simulink model "DCDC_SEPIC_TopLevelModel"  (R2024b)
settings: configuration reference "ConfigSet_ode23t_TopLevel" (kept outside this file)
undefined symbols (not defined in the file): psu_V, ts10ms, ts500us
libraries: fl_lib x21, ee_lib x9, dspstat3 x8, nesl_utility x7, simulink x3, batteryecm_lib x3, SEPIC_utilities x1
settings Model: DataDictionary=LocalDataD_TopLevelModelData.sldd  SILPILSystemUnderTest=refmodels  ExtModeTrigDuration=8  Creator=vivekr  LastModifiedBy=vlenzi
settings ConfigSetRef: SourceName=ConfigSet_ode23t_TopLevel

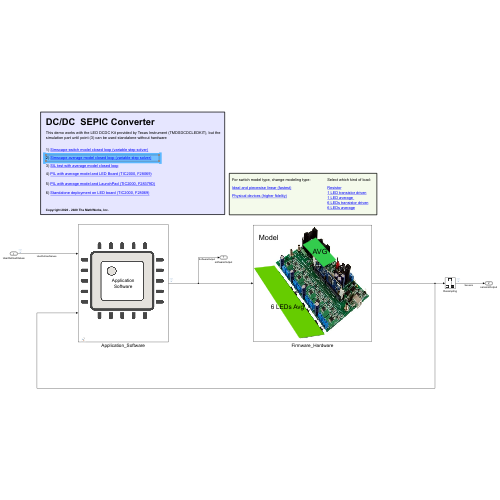
[thumbnail: Simulink's stored preview of the top-level diagram]
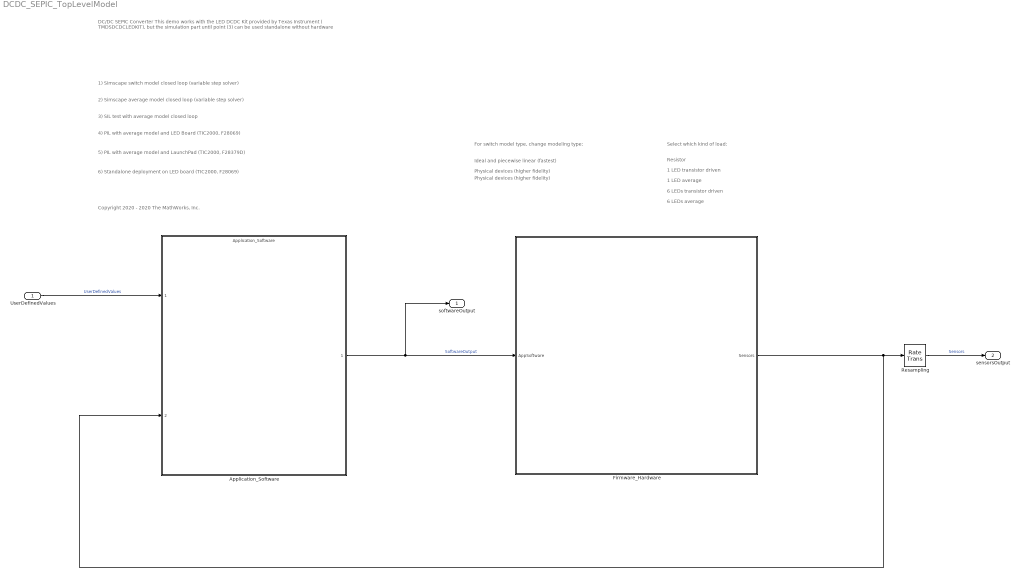
== system DCDC_SEPIC_TopLevelModel ==
  note: Copyright 2020 - 2020 The MathWorks, Inc.
  note: Ideal and piecewise linear (fastest)
  note: DC/DC SEPIC Converter
      |
      | This demo works with the LED DCDC Kit provided by Texas Instrument ( TMDSDCDCLEDKIT), but the simulation part until point (3) can be used standalone without hardware
  note: 6) Standalone deployment on LED board (TIC2000, F28069)
  note: 2) Simscape average model closed loop (variable step solver)
  note: 1) Simscape switch model closed loop (variable step solver)
  note: Physical devices (higher fidelity)
  note: For switch model type, change modeling type:
  note: 3) SIL test with average model closed loop
  note: Select which kind of load:
  note: Resistor
  note: 1 LED transistor driven
  note: 1 LED average
  note: 6 LEDs transistor driven
  note: 6 LEDs average
  note: 4) PIL with average model and LED Board (TIC2000, F28069)
  note: Physical devices (higher fidelity)
  note: 5) PIL with average model and LaunchPad (TIC2000, F28379D)
  UserDefinedValues : Inport  OutDataTypeStr=Bus: UserDefinedValues  Interpolate=off
  Application_Software : ModelReference  ModelNameDialog=Application_Software  SimulationMode=Normal  ModelReferenceVersion=9.13
      mask Display: image('cpu.png');disp('Application\nSoftware');
  Firmware_Hardware : Subsystem
      mask Display: image('SEPIC_converter_TI_Kit.jpg');patch([0.42 0.53 0.7 0.595],[0.83 0.89 0.7 0.64], [0.2 0.8 0.3]);text(0.505,0.78,'\fontsize{28}AVG','texmode', 'on');text(0.05,0.9,'\fontsize{28}Model','texmode', 'on');patch([0.39 0.01 0.18 0.6],[0.03 0.63 0.65 0.06], [0.4 0.8 0]);text(0.15,0.3,'\fontsize{25}6 LEDs Avg','texmode', 'on');
  Resampling : RateTransition  OutPortSampleTime=ts500us
  softwareOutput : Outport  OutDataTypeStr=Bus: AppSoftware
  sensorsOutput : Outport  Port=2  OutDataTypeStr=Bus: Sensors
  wires:
  Application_Software/1 -> Firmware_Hardware/1(AppSoftware), softwareOutput/1  "SoftwareOutput"
  Firmware_Hardware/1(Sensors) -> Resampling/1, Application_Software/2
  UserDefinedValues/1 -> Application_Software/1  "UserDefinedValues"
  Resampling/1 -> sensorsOutput/1  "Sensors"

== system DCDC_SEPIC_TopLevelModel/Firmware_Hardware ==
  Bus Element In : Inport  PortName=AppSoftware  Element=dcpwmSEPIC
  Bus Element In1 : Inport  PortName=AppSoftware  Element=dcpwmLEDvector
  Hardware_Filter : Subsystem  Variant=on  VariantControl=Variant1  AllowZeroVariantControls=on
  Bus Element Out : Outport  PortName=Sensors  Element=voltSEPIC
  Bus Element Out1 : Outport  PortName=Sensors  Element=currSEPIC
  Bus Element Out2 : Outport  PortName=Sensors  Element=currLEDstrips
  Bus Element Out3 : Outport  PortName=Sensors  Element=voltPSU
  wires:
  Hardware_Filter/2(currSEPIC) -> Bus Element Out1/1  "currSEPIC"
  Hardware_Filter/3(currLEDstrips) -> Bus Element Out2/1  "currLEDstrips"
  Bus Element In1/1 -> Hardware_Filter/2(dcpwmLEDvector)
  Hardware_Filter/4(voltPSU) -> Bus Element Out3/1  "voltPSU"
  Hardware_Filter/1(voltSEPIC) -> Bus Element Out/1  "voltSEPIC"
  Bus Element In/1 -> Hardware_Filter/1(dcpwmSEPIC)

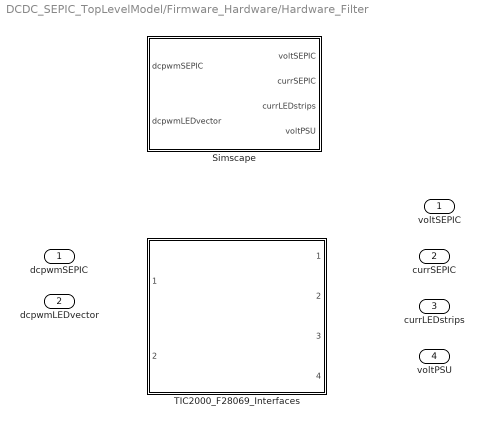
== system DCDC_SEPIC_TopLevelModel/Firmware_Hardware/Hardware_Filter ==
  dcpwmSEPIC : Inport  Unit=1
  dcpwmLEDvector : Inport  Port=2  Unit=1
  Simscape : Subsystem  VariantControl=Var_Plant==0
  TIC2000_F28069_Interfaces : Subsystem  VariantControl=Var_Plant ==1  ReferencedSubsystem=TIC2000_F28069_Interfaces
      settings: PermitHierarchicalResolution=None
  voltSEPIC : Outport  Unit=V  VectorParamsAs1DForOutWhenUnconnected=off
  currSEPIC : Outport  Port=2  Unit=mA  VectorParamsAs1DForOutWhenUnconnected=off
  currLEDstrips : Outport  Port=3  Unit=mA  PortDimensions=6  VectorParamsAs1DForOutWhenUnconnected=off
  voltPSU : Outport  Port=4  Unit=V  VectorParamsAs1DForOutWhenUnconnected=off

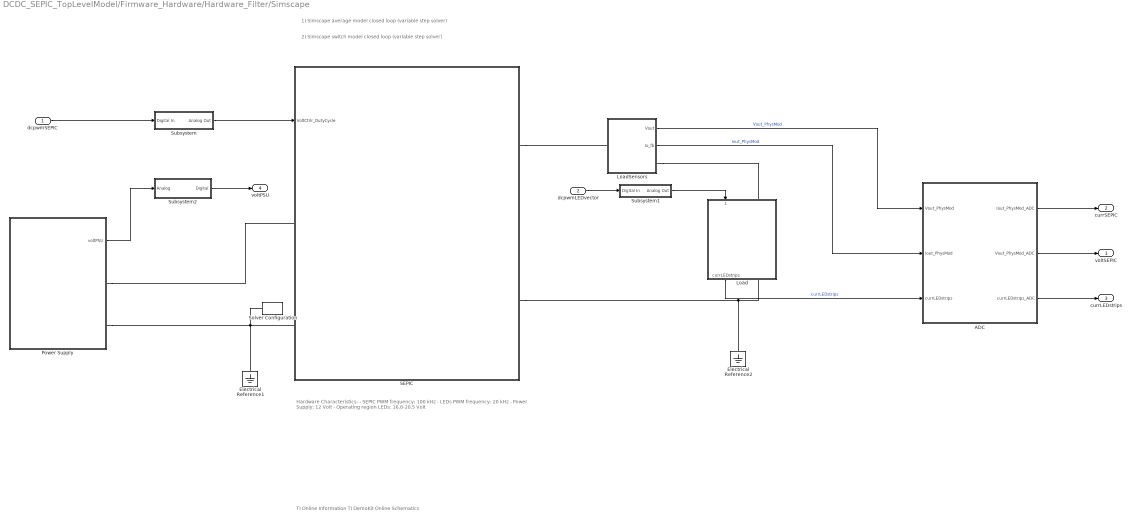
== system DCDC_SEPIC_TopLevelModel/Firmware_Hardware/Hardware_Filter/Simscape ==
  note: Hardware Characteristics:
      | - SEPIC PWM frequency: 100 kHz
      | - LEDs PWM frequency: 20 kHz
      | - Power Supply: 12 Volt
      | - Operating region LEDs: 16.8-20.5 Volt
  note: 2) Simscape switch model closed loop (variable step solver)
  note: 1) Simscape average model closed loop (variable step solver)
  note: TI Online Information
      | TI DemoKit Online Schematics
  dcpwmSEPIC : Inport  OutDataTypeStr=single  Unit=1  PortDimensions=1
  dcpwmLEDvector : Inport  Port=2  Unit=1
  ADC : Subsystem
      mask Display: disp('ADC');
  Electrical Reference1 : fl_lib/Electrical/Electrical Elements/Electrical Reference
  Electrical Reference2 : fl_lib/Electrical/Electrical Elements/Electrical Reference
  Load : Subsystem  Variant=on  VariantControlMode=label  VariantControl=Variant1  LabelModeActiveChoice=SixLEDStripsAvg
      mask Display: image('LED_Picture.jpg'); % Use "Edit Image" on toolstrip to change.
  LoadSensors : Subsystem
  Power Supply : Subsystem  Variant=on  VariantControlMode=label  VariantControl=Variant1  LabelModeActiveChoice=PowerSupply
      mask Display:
      | % Plot points to set plot range
      | color('white');plot(1.5, 2.5);plot(-1.5, -2)
      | color('black');
      | % Battery icon
      | plot([0 0], [2.5 1.3])
      | plot([0 0], [-0.6 -1.6])
      | patch([-1 1 1 -1]*0.4, [1 1 -1 -1]*0.15+0.7,[0;0;0]);
      | patch([-1 1 1 -1]*0.4, [1 1 -1 -1]*0.15-0.6,[0;0;0]);
      | patch([-1 1 1 -1]*0.8, [1 1 -1 -1]*0.15+1.3,[0;0;0]);
      | patch([-1 1 1 -1]*0.8, [1 1 -1 -1]*0.15+0.0,[0;0;0]);
      | text(1.2, 0.25,'+');
      | text(1.2,-1.1,'_');
      | text(1.2,1.8,'m');
  SEPIC : Subsystem  Variant=on  VariantControl=Variant1
      mask Display: image('dc_dc_converter.png'); % Use "Edit Image" on toolstrip to change.
  Solver Configuration : nesl_utility/Solver Configuration  PhysicalDomain=network_engine_domain  SubClassName=solver  LeftPortType=input  RightPortType=generic  Tones=[]  Harmonics=[]  SimulateNoise=off  Profile=off  UseLocalSampling=off  EnableSwitchedLinearOptims=on  FrequencyDomain=off  UseCCode=off  RelTol=0.001  AbsTol=1e-06  MinStep=1e-09  ToWorkspace=off  RevertToSquareIcSolve=off  NumHomotopyIterations=100  PhasorMode=off  PhasorModeNumHarmonics=1  ConsistencySolver=NEWTON_XTOL_AFTER_FTOL  IndexReductionMethod=DerivativeReplacement  DoDC=off  ResidualTolerance=1e-9  ConsistencyTolSource=GLOBAL  ConsistencyAbsTol=0.001  ConsistencyRelTol=0.001  ConsistencyTolFactor=0.001  UseLocalSolver=off  LocalSolverChoice=NE_BACKWARD_EULER_ADVANCER  ResolveIndetEquations=on  FunctionEvalNumThread=1  LocalSolverSampleTime=2e-7  DoFixedCost=off  MaxNonlinIter=2  MaxModeIter=2  ComputeImpulses=off  ImpulseIterations=2  LinearAlgebra=Sparse  LinearAlgebraNumThread=0  EquationFormulation=NE_TIME_EF  DelaysMemoryBudget=1024  AutomaticFiltering=on  FilteringTimeConstant=0.001  PartitionStorageMethod=AS_NEEDED  PartitionMemoryBudget=1024  PartitionMethod=ROBUST  MultibodyUseLocalSolver=off  MultibodyLocalSolverChoice=ODE1  MultibodyLocalSolverSampleTime=0.001
  Subsystem : Subsystem
      mask Display: disp('DAC')
  Subsystem1 : Subsystem
      mask Display: disp('DAC')
  Subsystem2 : Subsystem
      mask Display: disp('ADC')
  voltSEPIC : Outport  OutDataTypeStr=single  Unit=V  PortDimensions=1  VectorParamsAs1DForOutWhenUnconnected=off
  currSEPIC : Outport  Port=2  Unit=mA  VectorParamsAs1DForOutWhenUnconnected=off
  currLEDstrips : Outport  Port=3  Unit=mA  VectorParamsAs1DForOutWhenUnconnected=off
  voltPSU : Outport  Port=4  Unit=V  VectorParamsAs1DForOutWhenUnconnected=off
  wires:
  dcpwmLEDvector/1 -> Subsystem1/1(Digital In)
  LoadSensors/1(Vout) -> ADC/1(Vout_PhysMod)  "Vout_PhysMod"
  LoadSensors/2(Io_fb) -> ADC/2(Iout_PhysMod)  "Iout_PhysMod"
  Load/1(currLEDstrips) -> ADC/3(currLEDstrips)  "currLEDstrips"
  ADC/3(currLEDstrips_ADC) -> currLEDstrips/1
  ADC/2(Vout_PhysMod_ADC) -> voltSEPIC/1
  ADC/1(Iout_PhysMod_ADC) -> currSEPIC/1
  dcpwmSEPIC/1 -> Subsystem/1(Digital In)
  Subsystem/1(Analog Out) -> SEPIC/1(VoltCtrlr_DutyCycle)
  Subsystem1/1(Analog Out) -> Load/1(dcpwmLEDvector)
  Power Supply/1(voltPSU) -> Subsystem2/1(Analog)
  Subsystem2/1(Digital) -> voltPSU/1
  connections:
  LoadSensors/RConn1 -- Load/LConn1
  Electrical Reference2/LConn1 -- SEPIC/RConn2 -- Load/RConn1
  SEPIC/RConn1 -- LoadSensors/LConn1
  SEPIC/LConn2 -- Solver Configuration/RConn1 -- Electrical Reference1/LConn1 -- Power Supply/RConn2
  Power Supply/RConn1 -- SEPIC/LConn1

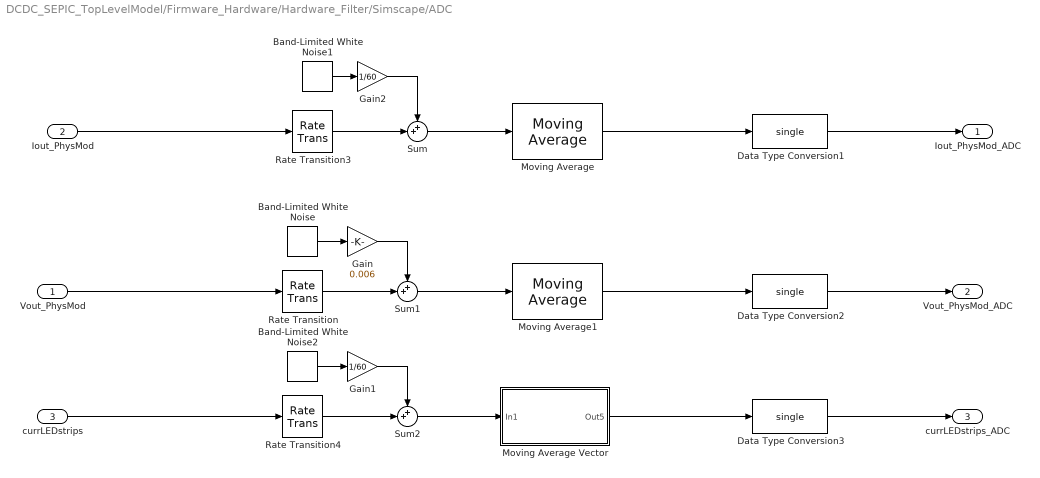
== system DCDC_SEPIC_TopLevelModel/Firmware_Hardware/Hardware_Filter/Simscape/ADC ==
  Vout_PhysMod : Inport
  Iout_PhysMod : Inport  Port=2
  currLEDstrips : Inport  Port=3
  Band-Limited White Noise : simulink/Sources/Band-Limited White Noise  Cov=0.1  Ts=ts500us  seed=[23341]
  Band-Limited White Noise1 : simulink/Sources/Band-Limited White Noise  Cov=2  Ts=ts10ms  seed=[23330]
  Band-Limited White Noise2 : simulink/Sources/Band-Limited White Noise  Cov=[2]  Ts=ts500us  seed=[23342]
  Data Type Conversion1 : DataTypeConversion  OutDataTypeStr=single  SaturateOnIntegerOverflow=off  RndMeth=Floor
  Data Type Conversion2 : DataTypeConversion  OutDataTypeStr=single  SaturateOnIntegerOverflow=off  RndMeth=Floor
  Data Type Conversion3 : DataTypeConversion  OutDataTypeStr=single  SaturateOnIntegerOverflow=off  RndMeth=Floor
  Gain : Gain  Gain=0.006
  Gain1 : Gain  Gain=1/60
  Gain2 : Gain  Gain=1/60
  Moving Average : dspstat3/Moving Average  Method=Exponential weighting  ForgettingFactorPort=off  SpecifyWindowLength=on  WindowLength=4  OverlapLength=3  AllowArbitraryInputLength=off  ForgettingFactor=0.93  SimulateUsing=Code generation
  Moving Average1 : dspstat3/Moving Average  Method=Exponential weighting  ForgettingFactorPort=off  SpecifyWindowLength=on  WindowLength=4  OverlapLength=3  AllowArbitraryInputLength=off  ForgettingFactor=0.93  SimulateUsing=Code generation
  Moving Average Vector : Subsystem
  Rate Transition : RateTransition  OutPortSampleTime=ts500us
  Rate Transition3 : RateTransition  OutPortSampleTime=ts10ms
  Rate Transition4 : RateTransition  OutPortSampleTime=ts500us
  Sum : Sum  Inputs=++|
  Sum1 : Sum  Inputs=++|
  Sum2 : Sum  Inputs=++|
  Iout_PhysMod_ADC : Outport
  Vout_PhysMod_ADC : Outport  Port=2
  currLEDstrips_ADC : Outport  Port=3
  wires:
  Vout_PhysMod/1 -> Rate Transition/1
  Data Type Conversion1/1 -> Iout_PhysMod_ADC/1
  Iout_PhysMod/1 -> Rate Transition3/1
  Moving Average/1 -> Data Type Conversion1/1
  currLEDstrips/1 -> Rate Transition4/1
  Data Type Conversion2/1 -> Vout_PhysMod_ADC/1
  Data Type Conversion3/1 -> currLEDstrips_ADC/1
  Rate Transition/1 -> Sum1/2
  Rate Transition3/1 -> Sum/2
  Rate Transition4/1 -> Sum2/2
  Band-Limited White Noise/1 -> Gain/1
  Band-Limited White Noise1/1 -> Gain2/1
  Band-Limited White Noise2/1 -> Gain1/1
  Sum/1 -> Moving Average/1
  Sum1/1 -> Moving Average1/1
  Moving Average1/1 -> Data Type Conversion2/1
  Gain/1 -> Sum1/1
  Gain1/1 -> Sum2/1
  Gain2/1 -> Sum/1
  Sum2/1 -> Moving Average Vector/1(In1)
  Moving Average Vector/1(Out5) -> Data Type Conversion3/1

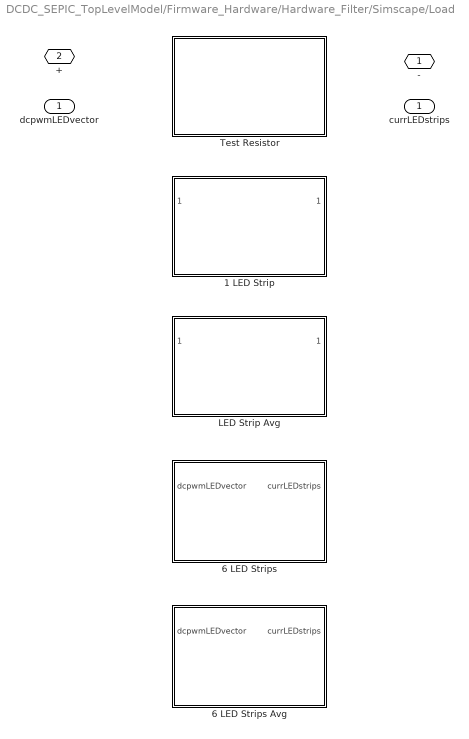
== system DCDC_SEPIC_TopLevelModel/Firmware_Hardware/Hardware_Filter/Simscape/Load ==
  dcpwmLEDvector : Inport
  1 LED Strip : Subsystem  VariantControl=SingleLEDStrip  ReferencedSubsystem=s1_LED_Strip
      settings: PermitHierarchicalResolution=None
  6 LED Strips : Subsystem  VariantControl=SixLEDStrips
  6 LED Strips Avg : Subsystem  VariantControl=SixLEDStripsAvg
  LED Strip Avg : Subsystem  VariantControl=SingleLEDStripAvg  ReferencedSubsystem=LED_Strip_Avg
      settings: PermitHierarchicalResolution=None
  Test Resistor : Subsystem  VariantControl=Resistor
  - : PMIOPort  Side=Right
  + : PMIOPort  Port=2  Side=Left
  currLEDstrips : Outport  Unit=mA  VectorParamsAs1DForOutWhenUnconnected=off

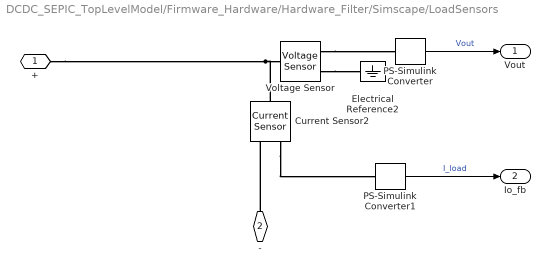
== system DCDC_SEPIC_TopLevelModel/Firmware_Hardware/Hardware_Filter/Simscape/LoadSensors ==
  Current Sensor2 : fl_lib/Electrical/Electrical Sensors/Current Sensor
  Electrical Reference2 : fl_lib/Electrical/Electrical Elements/Electrical Reference
  PS-Simulink Converter : nesl_utility/PS-Simulink Converter  PhysicalDomain=network_engine_domain  SubClassName=ps_output  LeftPortType=input  RightPortType=output  PseudoPeriodic=off  Frequencies=[]  VectorFormat=1-D array  Unit=V  AffineConversion=off
  PS-Simulink Converter1 : nesl_utility/PS-Simulink Converter  PhysicalDomain=network_engine_domain  SubClassName=ps_output  LeftPortType=input  RightPortType=output  PseudoPeriodic=off  Frequencies=[]  VectorFormat=1-D array  Unit=mA  AffineConversion=off
  Voltage Sensor : fl_lib/Electrical/Electrical Sensors/Voltage Sensor
  + : PMIOPort  Side=Left
  - : PMIOPort  Port=2  Side=Right
  Vout : Outport  VectorParamsAs1DForOutWhenUnconnected=off
  Io_fb : Outport  Port=2  VectorParamsAs1DForOutWhenUnconnected=off
  wires:
  PS-Simulink Converter1/1 -> Io_fb/1  "I_load"
  PS-Simulink Converter/1 -> Vout/1  "Vout"
  connections:
  Voltage Sensor/RConn1 -- PS-Simulink Converter/LConn1
  Voltage Sensor/RConn2 -- Electrical Reference2/LConn1
  Current Sensor2/LConn1 -- Voltage Sensor/LConn1 -- +/RConn1
  Current Sensor2/RConn1 -- PS-Simulink Converter1/LConn1
  -/RConn1 -- Current Sensor2/RConn2

== system DCDC_SEPIC_TopLevelModel/Firmware_Hardware/Hardware_Filter/Simscape/Power Supply ==
  Battery : Subsystem  VariantControl=Battery
      mask Display:
      | % Plot points to set plot range
      | color('white');plot(1.5, 2.5);plot(-1.5, -2)
      | color('black');
      | % Battery icon
      | plot([0 0], [2.5 1.3])
      | plot([0 0], [-0.6 -1.6])
      | patch([-1 1 1 -1]*0.4, [1 1 -1 -1]*0.15+0.7,[0;0;0]);
      | patch([-1 1 1 -1]*0.4, [1 1 -1 -1]*0.15-0.6,[0;0;0]);
      | patch([-1 1 1 -1]*0.8, [1 1 -1 -1]*0.15+1.3,[0;0;0]);
      | patch([-1 1 1 -1]*0.8, [1 1 -1 -1]*0.15+0.0,[0;0;0]);
      | text(1.2, 0.25,'+');
      | text(1.2,-1.1,'_');
      | text(1.2,1.8,'m');
  Power Supply : Subsystem  VariantControl=PowerSupply
  + : PMIOPort  Side=Right
  - : PMIOPort  Port=2  Side=Right
  voltPSU : Outport

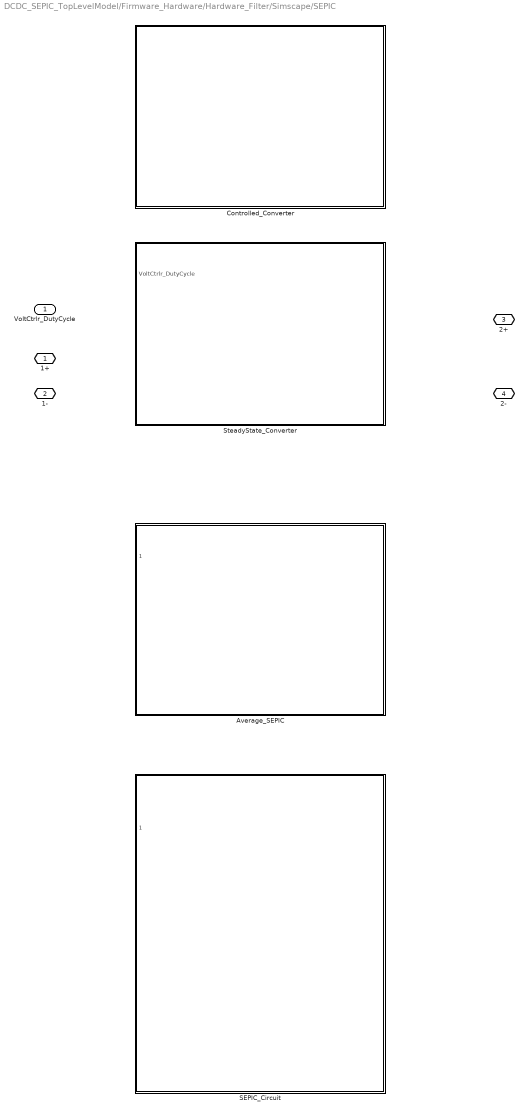
== system DCDC_SEPIC_TopLevelModel/Firmware_Hardware/Hardware_Filter/Simscape/SEPIC ==
  VoltCtrlr_DutyCycle : Inport
  Average_SEPIC : Subsystem  VariantControl=Var_Converter==3  ReferencedSubsystem=Average_SEPIC
      settings: PermitHierarchicalResolution=None
  Controlled_Converter : Subsystem  VariantControl=Var_Converter==0
  SEPIC_Circuit : Subsystem  VariantControl=Var_Converter==2  ReferencedSubsystem=SEPIC_Circuit
      settings: PermitHierarchicalResolution=None
  SteadyState_Converter : Subsystem  VariantControl=Var_Converter==1
  1+ : PMIOPort  Side=Left
  1- : PMIOPort  Port=2  Side=Left
  2+ : PMIOPort  Port=3  Side=Right
  2- : PMIOPort  Port=4  Side=Right

== system DCDC_SEPIC_TopLevelModel/Firmware_Hardware/Hardware_Filter/Simscape/Subsystem ==
  Digital In : Inport
  Data Type Conversion : DataTypeConversion  OutDataTypeStr=double  SaturateOnIntegerOverflow=off  RndMeth=Floor
  First Order Hold : FirstOrderHold  ErrorTolerance=inf
  Analog Out : Outport
  wires:
  First Order Hold/1 -> Analog Out/1  "dcpwmSEPIC"
  Data Type Conversion/1 -> First Order Hold/1
  Digital In/1 -> Data Type Conversion/1

== system DCDC_SEPIC_TopLevelModel/Firmware_Hardware/Hardware_Filter/Simscape/Subsystem1 ==
  Digital In : Inport
  Data Type Conversion : DataTypeConversion  OutDataTypeStr=double  SaturateOnIntegerOverflow=off  RndMeth=Floor
  First Order Hold : FirstOrderHold  ErrorTolerance=inf
  Analog Out : Outport
  wires:
  First Order Hold/1 -> Analog Out/1  "dcpwmSEPIC"
  Data Type Conversion/1 -> First Order Hold/1
  Digital In/1 -> Data Type Conversion/1

== system DCDC_SEPIC_TopLevelModel/Firmware_Hardware/Hardware_Filter/Simscape/Subsystem2 ==
  Analog : Inport
  Data Type Conversion4 : DataTypeConversion  OutDataTypeStr=single  SaturateOnIntegerOverflow=off  RndMeth=Floor
  Rate Transition3 : RateTransition  OutPortSampleTime=ts100ms
  Digital : Outport
  wires:
  Rate Transition3/1 -> Data Type Conversion4/1
  Data Type Conversion4/1 -> Digital/1
  Analog/1 -> Rate Transition3/1

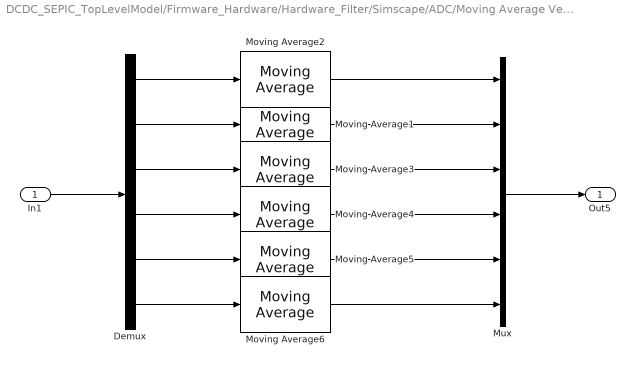
== system DCDC_SEPIC_TopLevelModel/Firmware_Hardware/Hardware_Filter/Simscape/ADC/Moving Average Vector ==
  In1 : Inport
  Demux : Demux  Outputs=6
  Moving Average{1..6} (6 alike) : dspstat3/Moving Average  Method=Exponential weighting  ForgettingFactorPort=off  SpecifyWindowLength=on  WindowLength=4  OverlapLength=3  AllowArbitraryInputLength=off  ForgettingFactor=0.93  SimulateUsing=Code generation
  Mux : Mux  Inputs=6
  Out5 : Outport
  wires:
  In1/1 -> Demux/1
  Moving Average2/1 -> Mux/1
  Demux/1 -> Moving Average2/1
  Demux/2 -> Moving Average1/1
  Demux/3 -> Moving Average3/1
  Demux/4 -> Moving Average4/1
  Demux/5 -> Moving Average5/1
  Demux/6 -> Moving Average6/1
  Moving Average1/1 -> Mux/2
  Moving Average3/1 -> Mux/3
  Moving Average4/1 -> Mux/4
  Moving Average5/1 -> Mux/5
  Moving Average6/1 -> Mux/6
  Mux/1 -> Out5/1

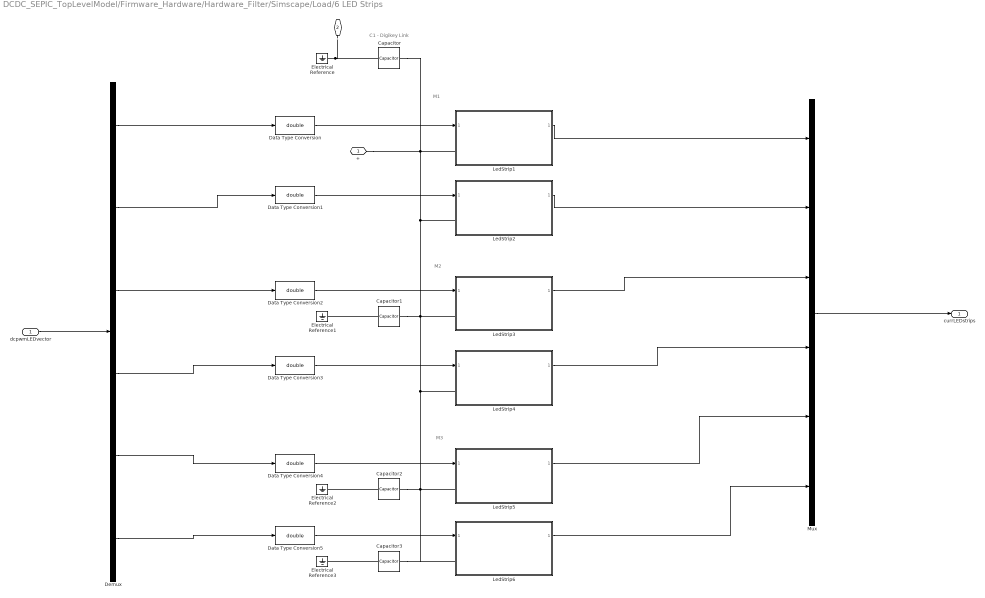
== system DCDC_SEPIC_TopLevelModel/Firmware_Hardware/Hardware_Filter/Simscape/Load/6 LED Strips ==
  note: M3
  note: M2
  note: M1
  note: C1 - Digikey Link
  dcpwmLEDvector : Inport
  Capacitor{,1..3} (4 alike) : ee_lib/Passive/Capacitor  cap_option=ee.enum.passive.capacitor.capOption.const  c=CLED_Cap uF  Cvec=[1e-05, 1e-06] F  Vvec=[0, 10] V  CV_table_symmetry=1  f_vec=[1, 10] kHz  DFext_vec=[.8, 1.2]  enable_C_tol=0  averaging_period=0 s  C_tol=CLED_Tol  tol_distribution=1  nSigma=4  r=CLED_Res Ohm  g=0 1/Ohm  enable_operating_limits=0  operating_limit_action=2  max_working_voltage_range=[-25, 25] V  power_rating=1 W  maxTemperature=85 degC  thermalEnable=false  thermalMass=1 J/K  fault_action=simscape.enum.assert.action.none  t_fault=1 s  i_specify=off  i_priority=None  i=0 A  i_nominal_specify=off  i_nominal_value=1  i_nominal_unit=A  v_specify=off  v_priority=None  v=0 V  v_nominal_specify=off  v_nominal_value=1  v_nominal_unit=V  vc_specify=off  vc_priority=High  vc=0 V  vc_nominal_specify=off  vc_nominal_value=1  vc_nominal_unit=V  T_specify=off  T_priority=None  T=298.15 K  T_nominal_specify=off  T_nominal_value=1  T_nominal_unit=K
  Data Type Conversion{,1..5} (6 alike) : DataTypeConversion  OutDataTypeStr=double  SaturateOnIntegerOverflow=off  RndMeth=Floor
  Demux : Demux  Outputs=6
  Electrical Reference{,1..3} (4 alike) : fl_lib/Electrical/Electrical Elements/Electrical Reference
  LedStrip{1..6} (6 alike) : Subsystem  ReferencedSubsystem=Subsystem_LEDStrip
      settings: PermitHierarchicalResolution=None
  Mux : Mux  Inputs=6
  + : PMIOPort  Side=Left
  - : PMIOPort  Port=2  Side=Right
  currLEDstrips : Outport  Unit=mA  VectorParamsAs1DForOutWhenUnconnected=off
  wires:
  Mux/1 -> currLEDstrips/1
  dcpwmLEDvector/1 -> Demux/1
  Demux/1 -> Data Type Conversion/1
  Data Type Conversion/1 -> LedStrip1/1
  LedStrip1/1 -> Mux/1
  Data Type Conversion1/1 -> LedStrip2/1
  LedStrip2/1 -> Mux/2
  LedStrip3/1 -> Mux/3
  LedStrip4/1 -> Mux/4
  LedStrip5/1 -> Mux/5
  LedStrip6/1 -> Mux/6
  Demux/2 -> Data Type Conversion1/1
  Demux/3 -> Data Type Conversion2/1
  Demux/4 -> Data Type Conversion3/1
  Demux/5 -> Data Type Conversion4/1
  Demux/6 -> Data Type Conversion5/1
  Data Type Conversion5/1 -> LedStrip6/1
  Data Type Conversion2/1 -> LedStrip3/1
  Data Type Conversion3/1 -> LedStrip4/1
  Data Type Conversion4/1 -> LedStrip5/1
  connections:
  Electrical Reference/LConn1 -- Capacitor/RConn1 -- -/RConn1
  +/RConn1 -- Capacitor/LConn1 -- Capacitor3/LConn1 -- LedStrip6/LConn1 -- Capacitor2/LConn1 -- LedStrip5/LConn1 -- LedStrip4/LConn1 -- Capacitor1/LConn1 -- LedStrip3/LConn1 -- LedStrip2/LConn1 -- LedStrip1/LConn1
  Capacitor1/RConn1 -- Electrical Reference1/LConn1
  Capacitor2/RConn1 -- Electrical Reference2/LConn1
  Capacitor3/RConn1 -- Electrical Reference3/LConn1

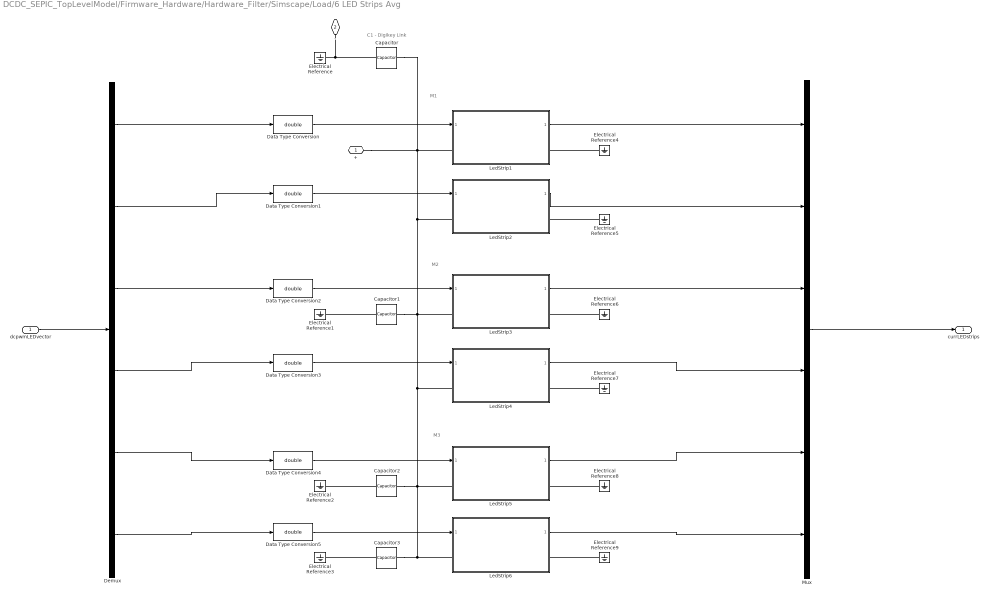
== system DCDC_SEPIC_TopLevelModel/Firmware_Hardware/Hardware_Filter/Simscape/Load/6 LED Strips Avg ==
  note: C1 - Digikey Link
  note: M1
  note: M2
  note: M3
  dcpwmLEDvector : Inport
  Capacitor{,1..3} (4 alike) : ee_lib/Passive/Capacitor  cap_option=ee.enum.passive.capacitor.capOption.const  c=CLED_Cap uF  Cvec=[1e-05, 1e-06] F  Vvec=[0, 10] V  CV_table_symmetry=1  f_vec=[1, 10] kHz  DFext_vec=[.8, 1.2]  enable_C_tol=0  averaging_period=0 s  C_tol=CLED_Tol  tol_distribution=1  nSigma=4  r=CLED_Res Ohm  g=0 1/Ohm  enable_operating_limits=0  operating_limit_action=2  max_working_voltage_range=[-25, 25] V  power_rating=1 W  maxTemperature=85 degC  thermalEnable=false  thermalMass=1 J/K  fault_action=simscape.enum.assert.action.none  t_fault=1 s  i_specify=off  i_priority=None  i=0 A  i_nominal_specify=off  i_nominal_value=1  i_nominal_unit=A  v_specify=off  v_priority=None  v=0 V  v_nominal_specify=off  v_nominal_value=1  v_nominal_unit=V  vc_specify=off  vc_priority=High  vc=0 V  vc_nominal_specify=off  vc_nominal_value=1  vc_nominal_unit=V  T_specify=off  T_priority=None  T=298.15 K  T_nominal_specify=off  T_nominal_value=1  T_nominal_unit=K
  Data Type Conversion{,1..5} (6 alike) : DataTypeConversion  OutDataTypeStr=double  SaturateOnIntegerOverflow=off  RndMeth=Floor
  Demux : Demux  Outputs=6
  Electrical Reference{,1..9} (10 alike) : fl_lib/Electrical/Electrical Elements/Electrical Reference
  LedStrip{1..6} (6 alike) : Subsystem  ReferencedSubsystem=Subsystem_LEDStripAvg
      settings: PermitHierarchicalResolution=None
  Mux : Mux  Inputs=6
  + : PMIOPort  Side=Left
  - : PMIOPort  Port=2  Side=Right
  currLEDstrips : Outport  Unit=mA  VectorParamsAs1DForOutWhenUnconnected=off
  wires:
  Data Type Conversion4/1 -> LedStrip5/1
  Data Type Conversion3/1 -> LedStrip4/1
  Data Type Conversion2/1 -> LedStrip3/1
  Data Type Conversion5/1 -> LedStrip6/1
  Demux/6 -> Data Type Conversion5/1
  Demux/5 -> Data Type Conversion4/1
  Demux/4 -> Data Type Conversion3/1
  Demux/3 -> Data Type Conversion2/1
  Demux/2 -> Data Type Conversion1/1
  LedStrip6/1 -> Mux/6
  LedStrip5/1 -> Mux/5
  LedStrip4/1 -> Mux/4
  LedStrip3/1 -> Mux/3
  LedStrip2/1 -> Mux/2
  Data Type Conversion1/1 -> LedStrip2/1
  LedStrip1/1 -> Mux/1
  Data Type Conversion/1 -> LedStrip1/1
  Demux/1 -> Data Type Conversion/1
  dcpwmLEDvector/1 -> Demux/1
  Mux/1 -> currLEDstrips/1
  connections:
  Capacitor3/RConn1 -- Electrical Reference3/LConn1
  Capacitor2/RConn1 -- Electrical Reference2/LConn1
  Capacitor1/RConn1 -- Electrical Reference1/LConn1
  Capacitor3/LConn1 -- LedStrip6/LConn1 -- LedStrip5/LConn1 -- LedStrip4/LConn1 -- LedStrip3/LConn1 -- LedStrip2/LConn1 -- LedStrip1/LConn1 -- +/RConn1 -- Capacitor/LConn1 -- Capacitor1/LConn1 -- Capacitor2/LConn1
  Capacitor/RConn1 -- -/RConn1 -- Electrical Reference/LConn1
  Electrical Reference4/LConn1 -- LedStrip1/RConn1
  Electrical Reference5/LConn1 -- LedStrip2/RConn1
  Electrical Reference6/LConn1 -- LedStrip3/RConn1
  Electrical Reference7/LConn1 -- LedStrip4/RConn1
  Electrical Reference8/LConn1 -- LedStrip5/RConn1
  Electrical Reference9/LConn1 -- LedStrip6/RConn1

== system DCDC_SEPIC_TopLevelModel/Firmware_Hardware/Hardware_Filter/Simscape/Load/Test Resistor ==
  Test Resistor : SEPIC_utilities/Test Resistor  VariantControl=Resistor  R_load=Rload_Res  R_tol=1
  - : PMIOPort  Side=Right
  + : PMIOPort  Port=2  Side=Left
  connections:
  Test Resistor/LConn1 -- +/RConn1
  Test Resistor/RConn1 -- -/RConn1

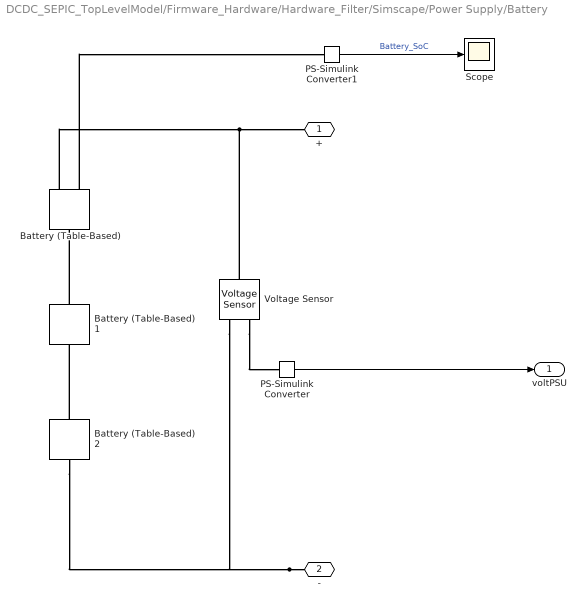
== system DCDC_SEPIC_TopLevelModel/Firmware_Hardware/Hardware_Filter/Simscape/Power Supply/Battery ==
  Battery (Table-Based) : batteryecm_lib/Battery (Table-Based)  SOC_vec=Batt_SoC_LUT  T_dependence=simscape.enum.tablebattery.temperature_dependence.no  prm_dir=simscape.enum.tablebattery.prm_dir.noCurrentDirectionality  T_vec=[273.15, 298.15, 323.15] K  V0_mat=[3.2, 3.1, 3.14; 3.25, 3.27, 3.3; 3.28, 3.31, 3.34; 3.33, 3.5, 3.59] V  V0_vec=Batt_Em0_LUT V  V_range=[0, inf] V  R0_mat=[.03, .015, .002; .04, .017, .008; .039, .012, .006; .027, .013, .021] Ohm  R0_vec=Batt_R0 Ohm  R0_dis_mat=[.03, .015, .002; .04, .017, .008; .039, .012, .006; .027, .013, .021] Ohm  R0_dis_vec=[.015, .017, .012, .013] Ohm  R0_ch_mat=[.03, .015, .002; .04, .017, .008; .039, .012, .006; .027, .013, .021] Ohm  R0_ch_vec=[.015, .017, .012, .013] Ohm  AH=Batt_Capacity hr*A  prm_leak=simscape.enum.tablebattery.prm_leak.disabled  Rleak_vec=[8000, 7000, 6000] Ohm  Rleak=7e3 Ohm  extrapolation_option=simscape.enum.extrapolation.linear  SOC_port=simscape.enum.tablebattery.enable.yes  prm_dyn=simscape.enum.tablebattery.prm_dyn.rc1  R1_mat=[.089, .076, .01; .042, .022, .099; .019, .007, .002; .051, .043, .029] Ohm  R1_vec=Batt_R1 Ohm  tau1_mat=[44, 148, 235; 93, 110, 1000; 19, 27, 133; .5, 22, 3] s  tau1_vec=Batt_Tau1 s  R2_mat=[.014, .382, .407; .028, .006, .007; .014, .007, .006; .333, .956, .912] Ohm  R2_vec=[.382, .006, .007, .956] Ohm  tau2_mat=[1, 44, 5644; 11, 24, 506; 2, 14, 330; 3310, 13419, 30216] s  tau2_vec=[44, 24, 14, 13419] s  R3_mat=[.014, .382, .407; .028, .006, .007; .014, .007, .006; .333, .956, .912] Ohm  R3_vec=[.382, .006, .007, .956] Ohm  tau3_mat=[1, 44, 5644; 11, 24, 506; 2, 14, 330; 3310, 13419, 30216] s  tau3_vec=[44, 24, 14, 13419] s  R4_mat=[.014, .382, .407; .028, .006, .007; .014, .007, .006; .333, .956, .912] Ohm  R4_vec=[.382, .006, .007, .956] Ohm  tau4_mat=[1, 44, 5644; 11, 24, 506; 2, 14, 330; 3310, 13419, 30216] s  tau4_vec=[44, 24, 14, 13419] s  R5_mat=[.014, .382, .407; .028, .006, .007; .014, .007, .006; .333, .956, .912] Ohm  R5_vec=[.382, .006, .007, .956] Ohm  tau5_mat=[1, 44, 5644; 11, 24, 506; 2, 14, 330; 3310, 13419, 30216] s  tau5_vec=[44, 24, 14, 13419] s  prm_fade=simscape.enum.tablebattery.prm_fade.equations  N0=100  dV0=0  dR0=0  dAH=0  dRleak=0  dR1=0  dR2=0  dR3=0  dR4=0  dR5=0  N0vec=[100, 200, 300]  Tfadevec=[298.15, 323.15] K  dV0vec=[0, 0, 0]  dR0vec=[0, 0, 0]  dAHvec=[0, 0, 0]  dRleakvec=[0, 0, 0]  dR1vec=[0, 0, 0]  dR2vec=[0, 0, 0]  dR3vec=[0, 0, 0]  dR4vec=[0, 0, 0]  dR5vec=[0, 0, 0]  dV0mat=[0, 0; 0, 0; 0, 0]  dR0mat=[0, 0; 0, 0; 0, 0]  dAHmat=[0, 0; 0, 0; 0, 0]  dRleakmat=[0, 0; 0, 0; 0, 0]  dR1mat=[0, 0; 0, 0; 0, 0]  dR2mat=[0, 0; 0, 0; 0, 0]  dR3mat=[0, 0; 0, 0; 0, 0]  dR4mat=[0, 0; 0, 0; 0, 0]  dR5mat=[0, 0; 0, 0; 0, 0]  prm_age_modeling=simscape.enum.tablebattery.prm_age_modeling.equation  storage_dt_age_vec=[0] d  storage_T_age_vec=[273] K  prm_age_OCV=simscape.enum.tablebattery.prm_age_OCV.OCV  OCV_age=0.9  SOC_age=0.6  prm_age_resistance=simscape.enum.tablebattery.prm_age.disabled  OCV_scaling_age_resistance=2.2134e6  OCV_offset_age_resistance=1.632e6  temp_exp_age_resistance=0.515833569 V  t_exp_age_resistance=0.75  T_age_vec_resistance=[273.15, 298.15, 323.15] K  dt_age_vec_resistance=[90, 180, 270, 360] d  dR0_age_vec=[0, 0, 0]  t_meas_dR0_age=100 d  dR0_age_mat=[0, 0, 0; 0, 0, 0; 0, 0, 0; 0, 0, 0]  prm_age_capacity=simscape.enum.tablebattery.prm_age.disabled  OCV_scaling_age_capacity=1.5097e07  OCV_offset_age_capacity=8.3625e06  temp_exp_age_capacity=0.6011 V  t_exp_age_capacity=0.75  T_age_vec_capacity=[273.15, 298.15, 323.15] K  dt_age_vec_capacity=[90, 180, 270, 360] d  dAH_age_vec=[0, 0, 0]  t_meas_dAH_age=100 d  dAH_age_mat=[0, 0, 0; 0, 0, 0; 0, 0, 0; 0, 0, 0]  thermal_port=simscape.enum.thermaleffects.omit  temperature=298.15 K  thermal_mass=30000 J/K  i_specify=off  i_priority=None  i=0 A  i_nominal_specify=off  i_nominal_value=1  i_nominal_unit=A  v_specify=off  v_priority=None  v=0 V  v_nominal_specify=off  v_nominal_value=1  v_nominal_unit=V  stateOfCharge_specify=on  stateOfCharge_priority=High  stateOfCharge=Batt_Initial_SoC  stateOfCharge_nominal_specify=off  stateOfCharge_nominal_value=1  stateOfCharge_nominal_unit=1  num_cycles_specify=off  num_cycles_priority=High  num_cycles=0  num_cycles_nominal_specify=off  num_cycles_nominal_value=1  num_cycles_nominal_unit=1  cell_temperature_specify=off  cell_temperature_priority=High  cell_temperature=298.15 K  cell_temperature_nominal_specify=off  cell_temperature_nominal_value=1  cell_temperature_nominal_unit=K
      settings: InternalSimscapePortConfiguration="{\"Bottom\":[],\"Left\":[{\"id\":\"p\",\"label\":\"+\",\"type\":\"foundation.electrical.electrical\"},{\"id\":\"soc\",\"label\":\"SOC\",\"type\":\"output\"}],\"Right\":[{\"id\":\"n\",\"label\":\"-\",\"type\":\"foundation.electrical.electrical\"}],\"Top\":[]}"
  Battery (Table-Based)1 : batteryecm_lib/Battery (Table-Based)  SOC_vec=Batt_SoC_LUT  T_dependence=simscape.enum.tablebattery.temperature_dependence.no  prm_dir=simscape.enum.tablebattery.prm_dir.noCurrentDirectionality  T_vec=[273.15, 298.15, 323.15] K  V0_mat=[3.2, 3.1, 3.14; 3.25, 3.27, 3.3; 3.28, 3.31, 3.34; 3.33, 3.5, 3.59] V  V0_vec=Batt_Em0_LUT V  V_range=[0, inf] V  R0_mat=[.03, .015, .002; .04, .017, .008; .039, .012, .006; .027, .013, .021] Ohm  R0_vec=Batt_R0 Ohm  R0_dis_mat=[.03, .015, .002; .04, .017, .008; .039, .012, .006; .027, .013, .021] Ohm  R0_dis_vec=[.015, .017, .012, .013] Ohm  R0_ch_mat=[.03, .015, .002; .04, .017, .008; .039, .012, .006; .027, .013, .021] Ohm  R0_ch_vec=[.015, .017, .012, .013] Ohm  AH=Batt_Capacity hr*A  prm_leak=simscape.enum.tablebattery.prm_leak.disabled  Rleak_vec=[8000, 7000, 6000] Ohm  Rleak=7e3 Ohm  extrapolation_option=simscape.enum.extrapolation.linear  SOC_port=simscape.enum.tablebattery.enable.no  prm_dyn=simscape.enum.tablebattery.prm_dyn.rc1  R1_mat=[.089, .076, .01; .042, .022, .099; .019, .007, .002; .051, .043, .029] Ohm  R1_vec=Batt_R1 Ohm  tau1_mat=[44, 148, 235; 93, 110, 1000; 19, 27, 133; .5, 22, 3] s  tau1_vec=Batt_Tau1 s  R2_mat=[.014, .382, .407; .028, .006, .007; .014, .007, .006; .333, .956, .912] Ohm  R2_vec=[.382, .006, .007, .956] Ohm  tau2_mat=[1, 44, 5644; 11, 24, 506; 2, 14, 330; 3310, 13419, 30216] s  tau2_vec=[44, 24, 14, 13419] s  R3_mat=[.014, .382, .407; .028, .006, .007; .014, .007, .006; .333, .956, .912] Ohm  R3_vec=[.382, .006, .007, .956] Ohm  tau3_mat=[1, 44, 5644; 11, 24, 506; 2, 14, 330; 3310, 13419, 30216] s  tau3_vec=[44, 24, 14, 13419] s  R4_mat=[.014, .382, .407; .028, .006, .007; .014, .007, .006; .333, .956, .912] Ohm  R4_vec=[.382, .006, .007, .956] Ohm  tau4_mat=[1, 44, 5644; 11, 24, 506; 2, 14, 330; 3310, 13419, 30216] s  tau4_vec=[44, 24, 14, 13419] s  R5_mat=[.014, .382, .407; .028, .006, .007; .014, .007, .006; .333, .956, .912] Ohm  R5_vec=[.382, .006, .007, .956] Ohm  tau5_mat=[1, 44, 5644; 11, 24, 506; 2, 14, 330; 3310, 13419, 30216] s  tau5_vec=[44, 24, 14, 13419] s  prm_fade=simscape.enum.tablebattery.prm_fade.equations  N0=100  dV0=0  dR0=0  dAH=0  dRleak=0  dR1=0  dR2=0  dR3=0  dR4=0  dR5=0  N0vec=[100, 200, 300]  Tfadevec=[298.15, 323.15] K  dV0vec=[0, 0, 0]  dR0vec=[0, 0, 0]  dAHvec=[0, 0, 0]  dRleakvec=[0, 0, 0]  dR1vec=[0, 0, 0]  dR2vec=[0, 0, 0]  dR3vec=[0, 0, 0]  dR4vec=[0, 0, 0]  dR5vec=[0, 0, 0]  dV0mat=[0, 0; 0, 0; 0, 0]  dR0mat=[0, 0; 0, 0; 0, 0]  dAHmat=[0, 0; 0, 0; 0, 0]  dRleakmat=[0, 0; 0, 0; 0, 0]  dR1mat=[0, 0; 0, 0; 0, 0]  dR2mat=[0, 0; 0, 0; 0, 0]  dR3mat=[0, 0; 0, 0; 0, 0]  dR4mat=[0, 0; 0, 0; 0, 0]  dR5mat=[0, 0; 0, 0; 0, 0]  prm_age_modeling=simscape.enum.tablebattery.prm_age_modeling.equation  storage_dt_age_vec=[0] d  storage_T_age_vec=[273] K  prm_age_OCV=simscape.enum.tablebattery.prm_age_OCV.OCV  OCV_age=0.9  SOC_age=0.6  prm_age_resistance=simscape.enum.tablebattery.prm_age.disabled  OCV_scaling_age_resistance=2.2134e6  OCV_offset_age_resistance=1.632e6  temp_exp_age_resistance=0.515833569 V  t_exp_age_resistance=0.75  T_age_vec_resistance=[273.15, 298.15, 323.15] K  dt_age_vec_resistance=[90, 180, 270, 360] d  dR0_age_vec=[0, 0, 0]  t_meas_dR0_age=100 d  dR0_age_mat=[0, 0, 0; 0, 0, 0; 0, 0, 0; 0, 0, 0]  prm_age_capacity=simscape.enum.tablebattery.prm_age.disabled  OCV_scaling_age_capacity=1.5097e07  OCV_offset_age_capacity=8.3625e06  temp_exp_age_capacity=0.6011 V  t_exp_age_capacity=0.75  T_age_vec_capacity=[273.15, 298.15, 323.15] K  dt_age_vec_capacity=[90, 180, 270, 360] d  dAH_age_vec=[0, 0, 0]  t_meas_dAH_age=100 d  dAH_age_mat=[0, 0, 0; 0, 0, 0; 0, 0, 0; 0, 0, 0]  thermal_port=simscape.enum.thermaleffects.omit  temperature=298.15 K  thermal_mass=30000 J/K  i_specify=off  i_priority=None  i=0 A  i_nominal_specify=off  i_nominal_value=1  i_nominal_unit=A  v_specify=off  v_priority=None  v=0 V  v_nominal_specify=off  v_nominal_value=1  v_nominal_unit=V  stateOfCharge_specify=on  stateOfCharge_priority=High  stateOfCharge=Batt_Initial_SoC  stateOfCharge_nominal_specify=off  stateOfCharge_nominal_value=1  stateOfCharge_nominal_unit=1  num_cycles_specify=off  num_cycles_priority=High  num_cycles=0  num_cycles_nominal_specify=off  num_cycles_nominal_value=1  num_cycles_nominal_unit=1  cell_temperature_specify=off  cell_temperature_priority=High  cell_temperature=298.15 K  cell_temperature_nominal_specify=off  cell_temperature_nominal_value=1  cell_temperature_nominal_unit=K
      settings: InternalSimscapePortConfiguration="{\"Bottom\":[],\"Left\":[{\"id\":\"p\",\"label\":\"+\",\"type\":\"foundation.electrical.electrical\"}],\"Right\":[{\"id\":\"n\",\"label\":\"-\",\"type\":\"foundation.electrical.electrical\"}],\"Top\":[]}"
  Battery (Table-Based)2 : batteryecm_lib/Battery (Table-Based)  SOC_vec=Batt_SoC_LUT  T_dependence=simscape.enum.tablebattery.temperature_dependence.no  prm_dir=simscape.enum.tablebattery.prm_dir.noCurrentDirectionality  T_vec=[273.15, 298.15, 323.15] K  V0_mat=[3.2, 3.1, 3.14; 3.25, 3.27, 3.3; 3.28, 3.31, 3.34; 3.33, 3.5, 3.59] V  V0_vec=Batt_Em0_LUT V  V_range=[0, inf] V  R0_mat=[.03, .015, .002; .04, .017, .008; .039, .012, .006; .027, .013, .021] Ohm  R0_vec=Batt_R0 Ohm  R0_dis_mat=[.03, .015, .002; .04, .017, .008; .039, .012, .006; .027, .013, .021] Ohm  R0_dis_vec=[.015, .017, .012, .013] Ohm  R0_ch_mat=[.03, .015, .002; .04, .017, .008; .039, .012, .006; .027, .013, .021] Ohm  R0_ch_vec=[.015, .017, .012, .013] Ohm  AH=Batt_Capacity hr*A  prm_leak=simscape.enum.tablebattery.prm_leak.disabled  Rleak_vec=[8000, 7000, 6000] Ohm  Rleak=7e3 Ohm  extrapolation_option=simscape.enum.extrapolation.linear  SOC_port=simscape.enum.tablebattery.enable.no  prm_dyn=simscape.enum.tablebattery.prm_dyn.rc1  R1_mat=[.089, .076, .01; .042, .022, .099; .019, .007, .002; .051, .043, .029] Ohm  R1_vec=Batt_R1 Ohm  tau1_mat=[44, 148, 235; 93, 110, 1000; 19, 27, 133; .5, 22, 3] s  tau1_vec=Batt_Tau1 s  R2_mat=[.014, .382, .407; .028, .006, .007; .014, .007, .006; .333, .956, .912] Ohm  R2_vec=[.382, .006, .007, .956] Ohm  tau2_mat=[1, 44, 5644; 11, 24, 506; 2, 14, 330; 3310, 13419, 30216] s  tau2_vec=[44, 24, 14, 13419] s  R3_mat=[.014, .382, .407; .028, .006, .007; .014, .007, .006; .333, .956, .912] Ohm  R3_vec=[.382, .006, .007, .956] Ohm  tau3_mat=[1, 44, 5644; 11, 24, 506; 2, 14, 330; 3310, 13419, 30216] s  tau3_vec=[44, 24, 14, 13419] s  R4_mat=[.014, .382, .407; .028, .006, .007; .014, .007, .006; .333, .956, .912] Ohm  R4_vec=[.382, .006, .007, .956] Ohm  tau4_mat=[1, 44, 5644; 11, 24, 506; 2, 14, 330; 3310, 13419, 30216] s  tau4_vec=[44, 24, 14, 13419] s  R5_mat=[.014, .382, .407; .028, .006, .007; .014, .007, .006; .333, .956, .912] Ohm  R5_vec=[.382, .006, .007, .956] Ohm  tau5_mat=[1, 44, 5644; 11, 24, 506; 2, 14, 330; 3310, 13419, 30216] s  tau5_vec=[44, 24, 14, 13419] s  prm_fade=simscape.enum.tablebattery.prm_fade.equations  N0=100  dV0=0  dR0=0  dAH=0  dRleak=0  dR1=0  dR2=0  dR3=0  dR4=0  dR5=0  N0vec=[100, 200, 300]  Tfadevec=[298.15, 323.15] K  dV0vec=[0, 0, 0]  dR0vec=[0, 0, 0]  dAHvec=[0, 0, 0]  dRleakvec=[0, 0, 0]  dR1vec=[0, 0, 0]  dR2vec=[0, 0, 0]  dR3vec=[0, 0, 0]  dR4vec=[0, 0, 0]  dR5vec=[0, 0, 0]  dV0mat=[0, 0; 0, 0; 0, 0]  dR0mat=[0, 0; 0, 0; 0, 0]  dAHmat=[0, 0; 0, 0; 0, 0]  dRleakmat=[0, 0; 0, 0; 0, 0]  dR1mat=[0, 0; 0, 0; 0, 0]  dR2mat=[0, 0; 0, 0; 0, 0]  dR3mat=[0, 0; 0, 0; 0, 0]  dR4mat=[0, 0; 0, 0; 0, 0]  dR5mat=[0, 0; 0, 0; 0, 0]  prm_age_modeling=simscape.enum.tablebattery.prm_age_modeling.equation  storage_dt_age_vec=[0] d  storage_T_age_vec=[273] K  prm_age_OCV=simscape.enum.tablebattery.prm_age_OCV.OCV  OCV_age=0.9  SOC_age=0.6  prm_age_resistance=simscape.enum.tablebattery.prm_age.disabled  OCV_scaling_age_resistance=2.2134e6  OCV_offset_age_resistance=1.632e6  temp_exp_age_resistance=0.515833569 V  t_exp_age_resistance=0.75  T_age_vec_resistance=[273.15, 298.15, 323.15] K  dt_age_vec_resistance=[90, 180, 270, 360] d  dR0_age_vec=[0, 0, 0]  t_meas_dR0_age=100 d  dR0_age_mat=[0, 0, 0; 0, 0, 0; 0, 0, 0; 0, 0, 0]  prm_age_capacity=simscape.enum.tablebattery.prm_age.disabled  OCV_scaling_age_capacity=1.5097e07  OCV_offset_age_capacity=8.3625e06  temp_exp_age_capacity=0.6011 V  t_exp_age_capacity=0.75  T_age_vec_capacity=[273.15, 298.15, 323.15] K  dt_age_vec_capacity=[90, 180, 270, 360] d  dAH_age_vec=[0, 0, 0]  t_meas_dAH_age=100 d  dAH_age_mat=[0, 0, 0; 0, 0, 0; 0, 0, 0; 0, 0, 0]  thermal_port=simscape.enum.thermaleffects.omit  temperature=298.15 K  thermal_mass=30000 J/K  i_specify=off  i_priority=None  i=0 A  i_nominal_specify=off  i_nominal_value=1  i_nominal_unit=A  v_specify=off  v_priority=None  v=0 V  v_nominal_specify=off  v_nominal_value=1  v_nominal_unit=V  stateOfCharge_specify=on  stateOfCharge_priority=High  stateOfCharge=Batt_Initial_SoC  stateOfCharge_nominal_specify=off  stateOfCharge_nominal_value=1  stateOfCharge_nominal_unit=1  num_cycles_specify=off  num_cycles_priority=High  num_cycles=0  num_cycles_nominal_specify=off  num_cycles_nominal_value=1  num_cycles_nominal_unit=1  cell_temperature_specify=off  cell_temperature_priority=High  cell_temperature=298.15 K  cell_temperature_nominal_specify=off  cell_temperature_nominal_value=1  cell_temperature_nominal_unit=K
      settings: InternalSimscapePortConfiguration="{\"Bottom\":[],\"Left\":[{\"id\":\"p\",\"label\":\"+\",\"type\":\"foundation.electrical.electrical\"}],\"Right\":[{\"id\":\"n\",\"label\":\"-\",\"type\":\"foundation.electrical.electrical\"}],\"Top\":[]}"
  PS-Simulink Converter : nesl_utility/PS-Simulink Converter  PhysicalDomain=network_engine_domain  SubClassName=ps_output  LeftPortType=input  RightPortType=output  PseudoPeriodic=off  Frequencies=[]  VectorFormat=1-D array  Unit=V  AffineConversion=off
  PS-Simulink Converter1 : nesl_utility/PS-Simulink Converter  PhysicalDomain=network_engine_domain  SubClassName=ps_output  LeftPortType=input  RightPortType=output  PseudoPeriodic=off  Frequencies=[]  VectorFormat=1-D array  Unit=inherit  AffineConversion=off
  Scope : Scope
  Voltage Sensor : fl_lib/Electrical/Electrical Sensors/Voltage Sensor
  + : PMIOPort  Side=Right
  - : PMIOPort  Port=2  Side=Right
  voltPSU : Outport  Unit=V  VectorParamsAs1DForOutWhenUnconnected=off
  wires:
  PS-Simulink Converter/1 -> voltPSU/1
  PS-Simulink Converter1/1 -> Scope/1  "Battery_SoC"
  connections:
  Battery (Table-Based)/LConn1 -- Voltage Sensor/LConn1 -- +/RConn1
  Battery (Table-Based)1/LConn1 -- Battery (Table-Based)/RConn1
  Battery (Table-Based)2/LConn1 -- Battery (Table-Based)1/RConn1
  -/RConn1 -- Battery (Table-Based)2/RConn1 -- Voltage Sensor/RConn2
  Voltage Sensor/RConn1 -- PS-Simulink Converter/LConn1
  Battery (Table-Based)/LConn2 -- PS-Simulink Converter1/LConn1

== system DCDC_SEPIC_TopLevelModel/Firmware_Hardware/Hardware_Filter/Simscape/Power Supply/Power Supply ==
  Controlled Voltage Source : fl_lib/Electrical/Electrical Sources/Controlled Voltage Source
  Simulink-PS Converter : nesl_utility/Simulink-PS Converter  PhysicalDomain=network_engine_domain  SubClassName=ps_input  LeftPortType=input  RightPortType=output  PseudoPeriodic=off  Frequencies=[]  NoiseDistribution=none  NoiseParameters=[]  Unit=V  AffineConversion=off  FilteringAndDerivatives=provide  SimscapeFilterOrder=1  InputFilterTimeConstant=0.001  UdotUserProvided=0
  voltage PSU : Constant  Value=psu_V  OutDataTypeStr=double
  + : PMIOPort  Side=Right
  - : PMIOPort  Port=2  Side=Right
  voltPSU : Outport  Unit=V  VectorParamsAs1DForOutWhenUnconnected=off
  wires:
  voltage PSU/1 -> voltPSU/1, Simulink-PS Converter/1
  connections:
  Controlled Voltage Source/RConn2 -- -/RConn1
  Controlled Voltage Source/RConn1 -- Simulink-PS Converter/RConn1
  Controlled Voltage Source/LConn1 -- +/RConn1

== system DCDC_SEPIC_TopLevelModel/Firmware_Hardware/Hardware_Filter/Simscape/SEPIC/Controlled_Converter ==
  DC-DC Converter : ee_lib/Semiconductors & Converters/Converters/DC-DC Converter  Vref_option=ee.enum.converters.voltageref.internal  v_ref=20 V  P_rated=50 W  droop_enabled=true  droop_param=1  droop=0.1 V/A  droop_percent=2  Vref_droop=10 V  reversible=0  G_diode=1e-8 1/Ohm  P_fixed=1 W  losses_option=ee.enum.converters.lossesOption.proportionalToSquaredCurrent  eff_rated=80  tableOption=ee.enum.converters.lossTableOption.current  i_eff_vec=[1, 2, 3, 4] A  v_eff_vec=[15, 30, 45] V  eff_vec=[90, 80, 70, 60]  eff_2D_table=[90, 85, 80; 80, 75, 70; 70, 65, 60; 60, 55, 50]  model_dynamics=1  tau=0.01 s  v_ini=0 V  v1_min=1 V  R1=1000 Ohm  R2=1000 Ohm  fault_condition=1  fault_threshold=0.5  T_eff_vec=[280, 300, 320] K  eff_3D_table=repmat([66; 76; 80; 74], 1, 3, 3)  thermal_mass=100 J/K  initial_temperature=298.15 K
      settings: InternalSimscapePortConfiguration="{\"Bottom\":[],\"Left\":[{\"id\":\"p1\",\"label\":\"1+\",\"type\":\"foundation.electrical.electrical\"},{\"id\":\"n1\",\"label\":\"1-\",\"type\":\"foundation.electrical.electrical\"}],\"Right\":[{\"id\":\"p2\",\"label\":\"2+\",\"type\":\"foundation.electrical.electrical\"},{\"id\":\"n2\",\"label\":\"2-\",\"type\":\"foundation.electrical.electrical\"}],\"Top\":[]}"
  1+ : PMIOPort  Side=Left
  1- : PMIOPort  Port=2  Side=Left
  2+ : PMIOPort  Port=3  Side=Right
  2- : PMIOPort  Port=4  Side=Right
  connections:
  1-/RConn1 -- DC-DC Converter/LConn2
  1+/RConn1 -- DC-DC Converter/LConn1
  2-/RConn1 -- DC-DC Converter/RConn2
  2+/RConn1 -- DC-DC Converter/RConn1

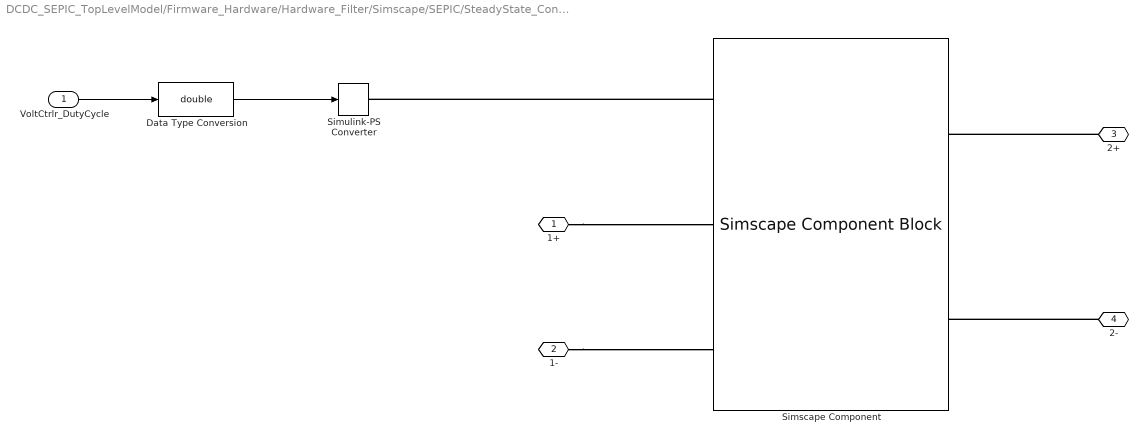
== system DCDC_SEPIC_TopLevelModel/Firmware_Hardware/Hardware_Filter/Simscape/SEPIC/SteadyState_Converter ==
  VoltCtrlr_DutyCycle : Inport
  Data Type Conversion : DataTypeConversion  OutDataTypeStr=double  SaturateOnIntegerOverflow=off  RndMeth=Floor
  Simscape Component : SimscapeComponentBlock  SourceFile=AverageSEPIC  ComponentPath=AverageSEPIC  ComponentVariants=AverageSEPIC  ComponentVariantNames=AverageSEPIC  ClassName=AverageSEPIC  SchemaVersion=1  i1_specify=off  i1_priority=None  i1=0 A  i1_nominal_specify=off  i1_nominal_value=1  i1_nominal_unit=A  v1_specify=off  v1_priority=None  v1=0 V  v1_nominal_specify=off  v1_nominal_value=1  v1_nominal_unit=V  i2_specify=off  i2_priority=None  i2=0 A  i2_nominal_specify=off  i2_nominal_value=1  i2_nominal_unit=A  v2_specify=off  v2_priority=None  v2=0 V  v2_nominal_specify=off  v2_nominal_value=1  v2_nominal_unit=V  n_specify=off  n_priority=None  n=1  n_nominal_specify=off  n_nominal_value=1  n_nominal_unit=1
      settings: CopyFcn=simscape.engine.sli.internal.componentblockcallback(gcbh,'COPY')  PreCopyFcn=simscape.engine.sli.internal.componentblockcallback(gcbh,'PRECOPY')  PreDeleteFcn=simscape.engine.sli.internal.componentblockcallback(gcbh,'PREDELETE')  InternalSimscapePortConfiguration="{\"Bottom\":[],\"Left\":[{\"id\":\"DC\",\"label\":\"dS\",\"type\":\"input\"},{\"id\":\"p1\",\"label\":\"1+\",\"type\":\"foundation.electrical.electrical\"},{\"id\":\"n1\",\"label\":\"1-\",\"type\":\"foundation.electrical.electrical\"}],\"Right\":[{\"id\":\"p2\",\"label\":\"2+\",\"type\":\"foundation.electrical.electrical\"},{\"id\":\"n2\",\"label\":\"2-\",\"type\":\"foundation.electrical.electrical\"}],\"Top\":[]}"
      mask Type: Average SEPIC model
  Simulink-PS Converter : nesl_utility/Simulink-PS Converter  PhysicalDomain=network_engine_domain  SubClassName=ps_input  LeftPortType=input  RightPortType=output  PseudoPeriodic=off  Frequencies=[]  NoiseDistribution=none  NoiseParameters=[]  Unit=1  AffineConversion=off  FilteringAndDerivatives=zero  SimscapeFilterOrder=1  InputFilterTimeConstant=0.001  UdotUserProvided=1
  1+ : PMIOPort  Side=Left
  1- : PMIOPort  Port=2  Side=Left
  2+ : PMIOPort  Port=3  Side=Right
  2- : PMIOPort  Port=4  Side=Right
  wires:
  Data Type Conversion/1 -> Simulink-PS Converter/1
  VoltCtrlr_DutyCycle/1 -> Data Type Conversion/1
  connections:
  2+/RConn1 -- Simscape Component/RConn1
  Simscape Component/LConn1 -- Simulink-PS Converter/RConn1
  1+/RConn1 -- Simscape Component/LConn2
  1-/RConn1 -- Simscape Component/LConn3
  2-/RConn1 -- Simscape Component/RConn2
